simulink model "fig_5_5"  (R2021b)
settings: Solver=ode23tb  StartTime=0.0  StopTime=1  FixedStep=1e-5  RelTol=1e-4  EnableMultiTasking=on
undefined symbols (not defined in the file): Ts
libraries: spsDiodeLib x4, spsSeriesRLCBranchLib x2, spsACVoltageSourceLib x1, spsLinearTransformerLib x1, spsMeanLib x1, spsMultimeterLib x1, spspowerguiLib x1
settings Model: Creator=umi  LastModifiedBy=DELL
settings SolverCC: AlgebraicLoopSolver=TrustRegion
settings DataIOCC: LimitDataPoints=on  SaveFormat=Array  ReturnWorkspaceOutputs=off
settings OptimizationCC: LifeSpan=inf
settings DebuggingCC: SolverPrmCheckMsg=warning  UnconnectedInputMsg=none  UnconnectedOutputMsg=none  UnconnectedLineMsg=none  SFUnexpectedBacktrackingDiag=warning  SFNoUnconditionalDefaultTransitionDiag=warning  SFExecutionAtInitializationDiag=none  SFMachineParentedDataDiag=warning  ArithmeticOperatorsInVariantConditions=warning
settings HardwareCC: ProdBitPerPointer=32  ProdBitPerSizeT=32  ProdBitPerPtrDiffT=32  ProdLargestAtomicFloat=None  ProdIntDivRoundTo=Undefined  ProdEndianess=Unspecified  ProdWordSize=32  ProdHWDeviceType=32-bit Generic
settings ModelReferenceCC: PropagateSignalLabelsOutOfModel=off
settings SFSimCC: SimUseLocalCustomCode=off  CustomCodeUndefinedFunction=UseInterfaceOnly
settings RTWCC: RTWUseLocalCustomCode=off
settings CodeAppCC: StateflowObjectComments=on
settings GRTTargetCC: TargetLangStandard=C89/C90 (ANSI)
settings ConfigComp: CovMetricSettings=dw  CovSaveCumulativeToWorkspaceVar=on  CovSaveSingleToWorkspaceVar=on  CovExternalEMLEnable=off  CovSFcnEnable=off
settings SimscapeCC: SimscapeNormalizeSystem=off

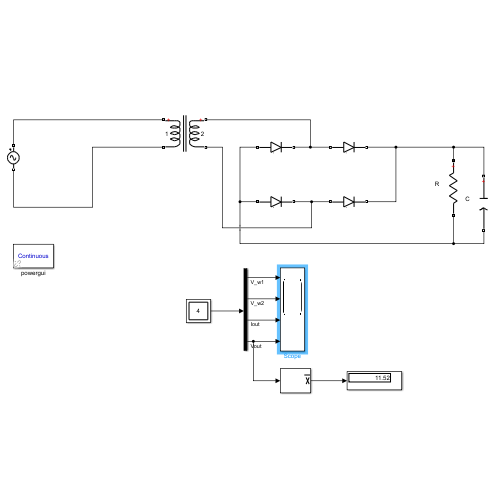
[thumbnail: Simulink's stored preview of the top-level diagram]
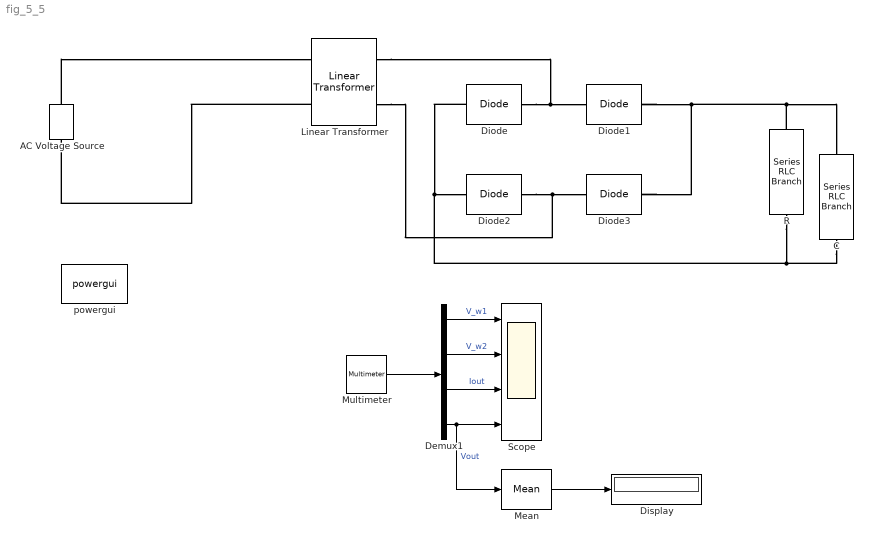
== system fig_5_5 ==
  AC Voltage Source : spsACVoltageSourceLib/AC Voltage Source  Amplitude=220*sqrt(2)  Phase=0  Frequency=50  SampleTime=0  Measurements=None  BusType=swing  Pref=10e3  Qref=0  Qmin=-inf  Qmax=+inf
  "C " : spsSeriesRLCBranchLib/Series RLC Branch  LConnTagsString=__new0  RConnTagsString=__new0  BranchType=C  Resistance=1  Inductance=1e-3  SetiL0=off  InitialCurrent=0  Capacitance=300e-6  Setx0=off  InitialVoltage=0  Measurements=Branch voltage
  Demux1 : Demux
  Diode{,1..3} (4 alike) : spsDiodeLib/Diode  Ron=0.05  Lon=1e-8  Vf=0.7  IC=0  UseSnubber=off  Rs=1e5  Cs=Inf  Measurements=off
  Display : Display
  Linear Transformer : spsLinearTransformerLib/Linear Transformer  UNITS=SI  NominalPower=[250e6 50]  winding1=[220 0 0]  winding2=[10 0 0]  ThreeWindings=off  winding3=[3.15e+05 0.7938 0.084223]  RmLm=[Inf 500e-6]  Measurements=Winding voltages  DataType=on
  Mean : spsMeanLib/Mean  Freq=50  Vinit=0  Ts=0
  Multimeter : spsMultimeterLib/Multimeter  PhasorSimulation=off  OutputType=Complex  sel=[2 3 4 1]  L=4  Gain=[1 1 1 1]  yselected={'Uw1: Linear Transformer','Uw2: Linear Transformer','Ib: R ','Ub: C '};  PSBOutputType=1  PSBequivalent=0  AxesSetting=[0,0.1,-100,100]  Display=0  SavedBlockNames=-11
  "R " : spsSeriesRLCBranchLib/Series RLC Branch  LConnTagsString=__new0  RConnTagsString=__new0  BranchType=R  Resistance=120  Inductance=1e-3  SetiL0=off  InitialCurrent=0  Capacitance=1e-6  Setx0=off  InitialVoltage=0  Measurements=Branch current
  Scope : Scope  NumInputPorts=4
  powergui : spspowerguiLib/powergui  Priority=1  SimulationMode=Continuous  SampleTime=Ts  frequency=60  Iterations=50  frequencyindice=0  Pbase=100e6  ErrMax=1e-4  UnitsV=kV  UnitsW=MW  buscounter=0  FunctionMessages=off  echomessages=off  EnableUseOfTLC=off  CurrentSourceSwitches=off  DisableSnubberDevices=on  DisableRonSwitches=off  DisableVfSwitches=off  DisplayEquations=off  AutomaticDiscreteSolvers=off  SolverType=Tustin/Backward Euler (TBE)  Interpol=off  ExternalGateDelay=off  methode=off  Ts=100  x0status=blocks  SPID=on  SwTol=0  HookPort=off  NonlinearTolerance=1e-4  nMaxIteration=100  ContinueOnMaxIteration=off  RestoreLinks=warning  ResistiveCurrentMeasurement=off  Frange=[0:2:500]  Ylog=off  Xlog=on  ShowGrid=off  save=off  variable=ZData  structure=0  ZoomFFT=off  StartTime=0.0  cycles=1  DisplayStyle=1  fundamental=60  FreqAxis=off  MaxFrequency=1000  frequencyindicesteady=1  RmsSteady=1  display=off
  wires:
  Mean/1 -> Display/1
  Multimeter/1 -> Demux1/1
  Demux1/1 -> Scope/1  "V_w1"
  Demux1/2 -> Scope/2  "V_w2"
  Demux1/3 -> Scope/3  "Iout"
  Demux1/4 -> Mean/1, Scope/4  "Vout"
  connections:
  AC Voltage Source/RConn1 -- Linear Transformer/LConn1
  "R "/LConn1 -- "C "/LConn1 -- Diode3/RConn1 -- Diode1/RConn1
  Linear Transformer/LConn2 -- AC Voltage Source/LConn1
  Diode2/RConn1 -- Linear Transformer/RConn2 -- Diode3/LConn1
  Diode/LConn1 -- "C "/RConn1 -- "R "/RConn1 -- Diode2/LConn1
  Diode/RConn1 -- Linear Transformer/RConn1 -- Diode1/LConn1
